simulink model "windturbine0x5B10x5D"  (R2024a)
settings: Solver=VariableStepAuto  StartTime=0.0  StopTime=10.0  RelTol=1e-3
libraries: spspowerguiLib x1
settings Model: Creator=ASUS  LastModifiedBy=ASUS

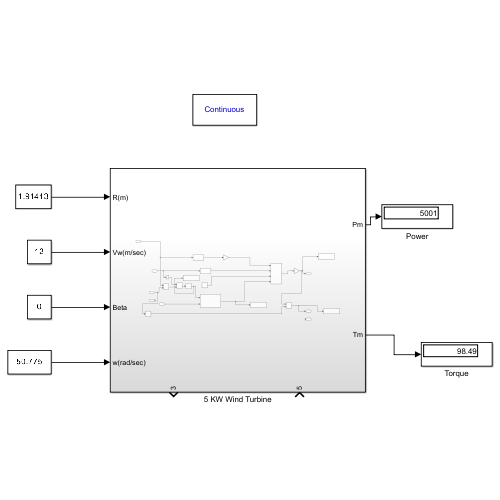
[thumbnail: Simulink's stored preview of the top-level diagram]
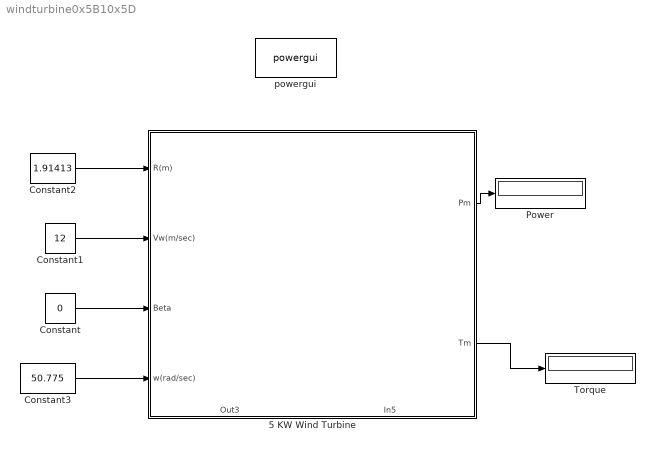
== system windturbine0x5B10x5D ==
  5 KW Wind Turbine : Subsystem
      settings: PortSchema="{\"entries\":[{\"content\":{\"sides\":[{\"content\":{\"connectorIds\":[\"In1\",\"In2\",\"In3\",\"In4\"]},\"type\":\"ConnectorPlacement.EquallySpacedRectSide\",\"uuid\":\"c135657b-e285-4412-802b-0a04abc77e6a\"},{\"content\":{\"connectorIds\":[\"Out1\",\"Out2\"],\"side\":\"RIGHT\"},\"type\":\"ConnectorPlacement.EquallySpacedRectSide\",\"uuid\":\"40798c73-7b02-41ba-b76b-de36934f1fa4\"},{\"content\":{\"side\":\"TOP\"},\"type\":\"ConnectorPlacement.EquallySpacedRectSide\",\"uuid\":\"7f505850-178c-4920-a9fb-b9b3bacb9a18\"},{\"content\":{\"connectorIds\":[\"Out3\",\"In5\"],\"side\":\"BOTTOM\"},\"type\":\"ConnectorPlacement.EquallySpacedRectSide\",\"uuid\":\"981118a8-62d9-4984-8d01-73a5da7afbd8\"}]},\"type\":\"ConnectorPlacement.EquallySpacedConnector\",\"uuid\":\"713ec3bb-dede-416f-9773-6b72b802f745\"}],\"packageUris\":[\"http://schema.mathworks.com/mf0/Connector/R2020b\"],\"version\":\"1.0\"}"
  Constant : Constant  Value=0
  Constant1 : Constant  Value=12
  Constant2 : Constant  Value=1.91413
  Constant3 : Constant  Value=50.775
  Power : Display
  Torque : Display
  powergui : spspowerguiLib/powergui  Priority=1  SimulationMode=Continuous  SampleTime=50e-6  frequency=60  Iterations=50  frequencyindice=60  Pbase=100e6  ErrMax=1e-4  UnitsV=kV  UnitsW=MW  buscounter=0  FunctionMessages=off  echomessages=off  EnableUseOfTLC=off  CurrentSourceSwitches=off  DisableSnubberDevices=off  DisableRonSwitches=off  DisableVfSwitches=off  DisplayEquations=off  AutomaticDiscreteSolvers=off  SolverType=Tustin/Backward Euler (TBE)  Interpol=off  ExternalGateDelay=off  methode=off  Ts=100  x0status=blocks  SPID=on  SwTol=0  HookPort=off  NonlinearTolerance=1e-4  nMaxIteration=100  ContinueOnMaxIteration=off  RestoreLinks=warning  ResistiveCurrentMeasurement=off  Frange=[0:2:500]  Ylog=off  Xlog=on  ShowGrid=off  save=off  variable=ZData  structure=0  ZoomFFT=off  StartTime=0.0  cycles=1  DisplayStyle=1  fundamental=60  FreqAxis=off  MaxFrequency=1000  frequencyindicesteady=1  RmsSteady=1  display=off
  wires:
  Constant/1 -> 5 KW Wind Turbine/3(Beta)
  Constant2/1 -> 5 KW Wind Turbine/1(R(m))
  Constant1/1 -> 5 KW Wind Turbine/2(Vw(m/sec))
  Constant3/1 -> 5 KW Wind Turbine/4(w(rad/sec))
  5 KW Wind Turbine/1(Pm) -> Power/1
  5 KW Wind Turbine/2(Tm) -> Torque/1

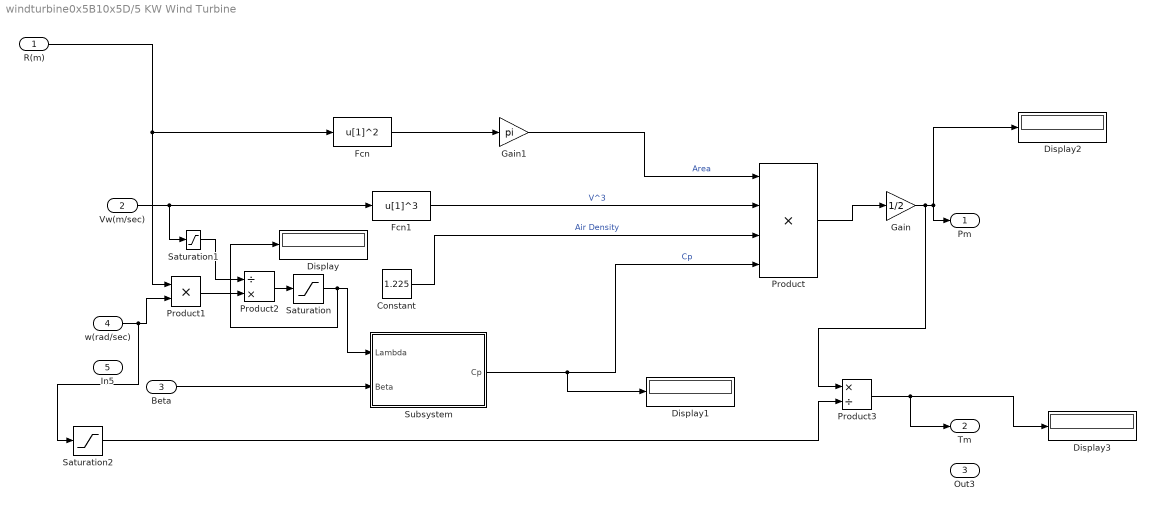
== system windturbine0x5B10x5D/5 KW Wind Turbine ==
  R(m) : Inport
  Vw(m/sec) : Inport  Port=2
  Beta : Inport  Port=3
  w(rad/sec) : Inport  Port=4
  In5 : Inport  Port=5
  Constant : Constant  Value=1.225
  Display{,1..3} (4 alike) : Display
  Fcn : Fcn  Expr=u[1]^2
  Fcn1 : Fcn  Expr=u[1]^3
  Gain : Gain  Gain=1/2
  Gain1 : Gain  Gain=pi
  Product : Product  Inputs=4
  Product1 : Product
  Product2 : Product  Inputs=/*
  Product3 : Product  Inputs=*/
  Saturation : Saturate  UpperLimit=inf  LowerLimit=1e-6
  Saturation1 : Saturate  UpperLimit=inf  LowerLimit=1e-6
  Saturation2 : Saturate  UpperLimit=inf  LowerLimit=1e-6
  Subsystem : Subsystem
  Pm : Outport
  Tm : Outport  Port=2
  Out3 : Outport  Port=3
  wires:
  Product/1 -> Gain/1
  Constant/1 -> Product/3  "Air Density"
  Subsystem/1(Cp) -> Display1/1, Product/4  "Cp"
  Fcn1/1 -> Product/2  "V^3"
  Gain1/1 -> Product/1  "Area"
  Fcn/1 -> Gain1/1
  R(m)/1 -> Product1/1, Fcn/1
  Vw(m/sec)/1 -> Fcn1/1, Saturation1/1
  Beta/1 -> Subsystem/2(Beta)
  w(rad/sec)/1 -> Saturation2/1, Product1/2
  Product1/1 -> Product2/2
  Product2/1 -> Saturation/1
  Saturation/1 -> Display/1, Subsystem/1(Lambda)
  Saturation1/1 -> Product2/1
  Saturation2/1 -> Product3/2
  Gain/1 -> Product3/1, Display2/1, Pm/1
  Product3/1 -> Display3/1, Tm/1

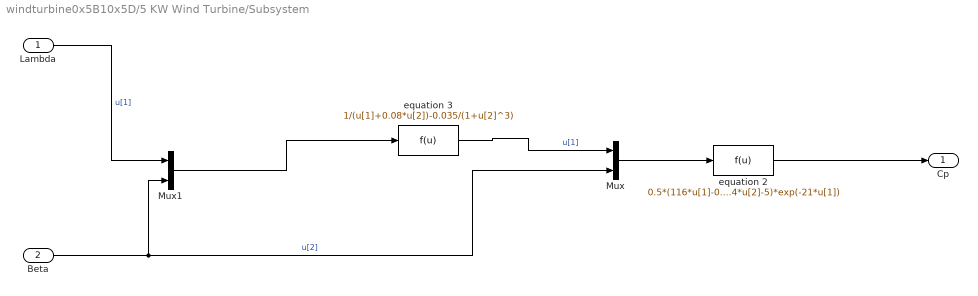
== system windturbine0x5B10x5D/5 KW Wind Turbine/Subsystem ==
  Lambda : Inport
  Beta : Inport  Port=2
  Mux : Mux  Inputs=2
  Mux1 : Mux  Inputs=2
  equation 2 : Fcn  Expr=0.5*(116*u[1]-0.4*u[2]-5)*exp(-21*u[1])
  equation 3 : Fcn  Expr=1/(u[1]+0.08*u[2])-0.035/(1+u[2]^3)
  Cp : Outport
  wires:
  equation 2/1 -> Cp/1
  Mux/1 -> equation 2/1
  Lambda/1 -> Mux1/1  "u[1]"
  equation 3/1 -> Mux/1  "u[1]"
  Beta/1 -> Mux/2, Mux1/2  "u[2]"
  Mux1/1 -> equation 3/1
